simulink library "sm_trackV_lib_terrain_contact"  (R2023b)
settings: Solver=VariableStepAuto  StartTime=0.0  StopTime=10.0  RelTol=1e-3
undefined symbols (not defined in the file): L1, L10, L11, L12, L13, L14, L15, L16, L17, L18, L19, L2, L20, L21, L22, L23, L24, L25, L26, L27, L28, L29, L3, L30, L31, L32, L33, L34, L35, L36, L37, L38, L39, L4, L40, L41, L42, L43, L44, L45, L46, L5, L6, L7, L8, L9, S1, S2, Scene
libraries: $bdroot x141, sm_lib x2
Description:
  | Copyright 2024 The MathWorks, Inc.
settings Model: Creator=smiller  LastModifiedBy=smiller

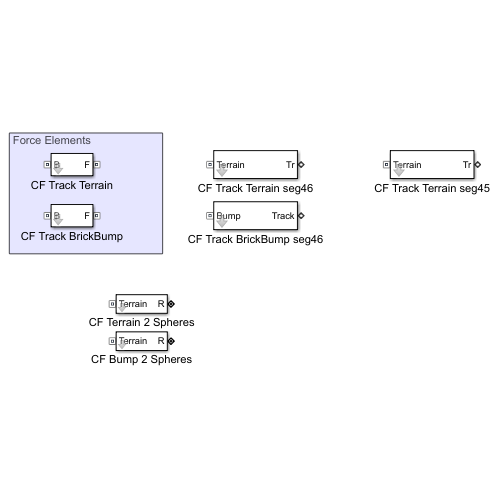
[thumbnail: Simulink's stored preview of the top-level diagram]
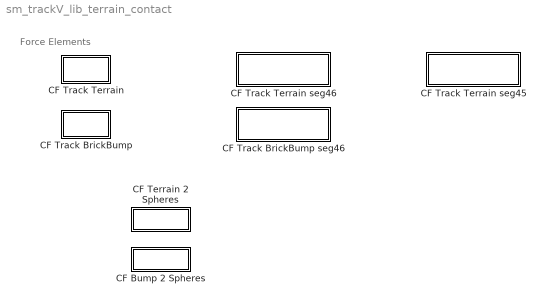
== system sm_trackV_lib_terrain_contact ==
  note: Force Elements
  CF Bump 2 Spheres : Subsystem  mask(Contact Force, Two Spheres to Bump){K_BrickBump=Scene.Contact.BrickBump.K, B_BrickBump=Scene.Contact.BrickBump.B, TW_BrickBump=Scene.Contact.BrickBump.TW, CoefficientOfDynamicFriction=Scene.Contact.Terrain.mud, CoefficientOfStaticFriction=Scene.Contact.Terrain.mus, FrictionalCriticalVelocity=Scene.Contact.Terrain.CV}
      mask prompts: K_BrickBump "Normal Stiffness (N/m)"; B_BrickBump "Normal Damping (N/(m/s))"; TW_BrickBump "Normal Transition Width (m)"; CoefficientOfDynamicFriction "Coefficient of Dynamic Friction"; CoefficientOfStaticFriction "Coefficient of Static Friction"; FrictionalCriticalVelocity "Critical Velocity (m/s)"
      mask help: Models contact force between two spheres and a bump.
      mask TypeOptions K_BrickBump: CF Bump Roller Sphere 1 /NormalStiffness | CF Bump Roller Sphere 2/NormalStiffness
      mask TypeOptions B_BrickBump: CF Bump Roller Sphere 1 /NormalDamping | CF Bump Roller Sphere 2/NormalDamping
      mask TypeOptions TW_BrickBump: CF Bump Roller Sphere 1 /NormalTransitionRegionWidth | CF Bump Roller Sphere 2/NormalTransitionRegionWidth
      mask TypeOptions CoefficientOfDynamicFriction: CF Bump Roller Sphere 1 /CoefficientOfDynamicFriction | CF Bump Roller Sphere 2/CoefficientOfDynamicFriction
      mask TypeOptions CoefficientOfStaticFriction: CF Bump Roller Sphere 1 /CoefficientOfStaticFriction | CF Bump Roller Sphere 2/CoefficientOfStaticFriction
      mask TypeOptions FrictionalCriticalVelocity: CF Bump Roller Sphere 1 /FrictionalCriticalVelocity | CF Bump Roller Sphere 2/FrictionalCriticalVelocity
  CF Terrain 2 Spheres : Subsystem  mask(Contact Force, Two Spheres to Ground){NormalStiffness=Scene.Contact.Spheres.Terrain.K, NormalDamping=Scene.Contact.Spheres.Terrain.B, NormalTransitionRegionWidth=Scene.Contact.Spheres.Terrain.TW, CoefficientOfDynamicFriction=Scene.Contact.Spheres.Terrain.mud, CoefficientOfStaticFriction=Scene.Contact.Spheres.Terrain.mus, FrictionalCriticalVelocity=Scene.Contact.Spheres.Terrain.CV}
      mask prompts: NormalStiffness "Normal Stiffness (N/m)"; NormalDamping "Normal Damping (N/(m/s))"; NormalTransitionRegionWidth "Normal Transition Width (m)"; CoefficientOfDynamicFriction "Coefficient of Dynamic Friction"; CoefficientOfStaticFriction "Coefficient of Static Friction"; FrictionalCriticalVelocity "Critical Velocity (m/s)"
      mask help: Models contact force between two spheres and the ground.
      mask TypeOptions NormalStiffness: CF Roller Sphere Terrain 1/NormalStiffness | CF Roller Sphere Terrain 2/NormalStiffness
      mask TypeOptions NormalDamping: CF Roller Sphere Terrain 1/NormalDamping | CF Roller Sphere Terrain 2/NormalDamping
      mask TypeOptions NormalTransitionRegionWidth: CF Roller Sphere Terrain 1/NormalTransitionRegionWidth | CF Roller Sphere Terrain 2/NormalTransitionRegionWidth
      mask TypeOptions CoefficientOfDynamicFriction: CF Roller Sphere Terrain 1/CoefficientOfDynamicFriction | CF Roller Sphere Terrain 2/CoefficientOfDynamicFriction
      mask TypeOptions CoefficientOfStaticFriction: CF Roller Sphere Terrain 1/CoefficientOfStaticFriction | CF Roller Sphere Terrain 2/CoefficientOfStaticFriction
      mask TypeOptions FrictionalCriticalVelocity: CF Roller Sphere Terrain 1/FrictionalCriticalVelocity | CF Roller Sphere Terrain 2/FrictionalCriticalVelocity
  CF Track BrickBump : Subsystem  mask(Contact Force, Track Segment to Bump){NormalStiffness=Scene.Contact.BrickBump.K, NormalDamping=Scene.Contact.BrickBump.B, NormalTransitionRegionWidth=Scene.Contact.BrickBump.TW}
      mask prompts: NormalStiffness "Normal Stiffness (N/m)"; NormalDamping "Normal Damping (N/(m/s))"; NormalTransitionRegionWidth "Normal Transition Width (m)"
      mask help: Models contact force between a track segment and a bump.
      mask TypeOptions NormalStiffness:
      | Spatial
      | Contact Force/NormalStiffness
      mask TypeOptions NormalDamping:
      | Spatial
      | Contact Force/NormalDamping
      mask TypeOptions NormalTransitionRegionWidth:
      | Spatial
      | Contact Force/NormalTransitionRegionWidth
  CF Track BrickBump seg46 : Subsystem  mask(Contact Forces, Full Track to Bump){K_BrickBump=Scene.Contact.BrickBump.K, B_BrickBump=Scene.Contact.BrickBump.B, TW_BrickBump=Scene.Contact.BrickBump.TW}
      mask prompts: K_BrickBump "Normal Stiffness (N/m)"; B_BrickBump "Normal Damping (N/(m/s))"; TW_BrickBump "Normal Transition Width (m)"
      mask help: Models contact force between all track segments and bump.
  CF Track Terrain : Subsystem  mask(Contact Force, Track Segment to Terrain){NormalStiffness=Scene.Contact.Terrain.K, NormalDamping=Scene.Contact.Terrain.B, NormalTransitionRegionWidth=Scene.Contact.Terrain.TW, CoefficientOfDynamicFriction=Scene.Contact.Terrain.mud, CoefficientOfStaticFriction=Scene.Contact.Terrain.mus, FrictionalCriticalVelocity=Scene.Contact.Terrain.CV}
      mask prompts: NormalStiffness "Normal Stiffness (N/m)"; NormalDamping "Normal Damping (N/(m/s))"; NormalTransitionRegionWidth "Normal Transition Width (m)"; CoefficientOfDynamicFriction "Coefficient of Dynamic Friction"; CoefficientOfStaticFriction "Coefficient of Static Friction"; FrictionalCriticalVelocity "Critical Velocity (m/s)"
      mask help: Models contact force between one track segment and the terrain.
      mask TypeOptions NormalStiffness:
      | Spatial
      | Contact Force/NormalStiffness
      mask TypeOptions NormalDamping:
      | Spatial
      | Contact Force/NormalDamping
      mask TypeOptions NormalTransitionRegionWidth:
      | Spatial
      | Contact Force/NormalTransitionRegionWidth
      mask TypeOptions CoefficientOfDynamicFriction:
      | Spatial
      | Contact Force/CoefficientOfDynamicFriction
      mask TypeOptions CoefficientOfStaticFriction:
      | Spatial
      | Contact Force/CoefficientOfStaticFriction
      mask TypeOptions FrictionalCriticalVelocity:
      | Spatial
      | Contact Force/FrictionalCriticalVelocity
  CF Track Terrain seg45 : Subsystem  mask(Contact Forces, Full Track to Terrain){K_Road=Scene.Contact.Terrain.K, B_Road=Scene.Contact.Terrain.B, TW_Road=Scene.Contact.Terrain.TW, F_dyn_Road=Scene.Contact.Terrain.mud, F_stat_Road=Scene.Contact.Terrain.mus, CV_Road=Scene.Contact.Terrain.CV}
      mask prompts: K_Road "Normal Stiffness (N/m)"; B_Road "Normal Damping (N/(m/s))"; TW_Road "Normal Transition Width (m)"; F_dyn_Road "Coefficient of Dynamic Friction"; F_stat_Road "Coefficient of Static Friction"; CV_Road "Critical Velocity (m/s)"
      mask help: Models contact force between all track segments and the terrain.
  CF Track Terrain seg46 : Subsystem  mask(Contact Forces, Full Track to Terrain){K_Road=Scene.Contact.Terrain.K, B_Road=Scene.Contact.Terrain.B, TW_Road=Scene.Contact.Terrain.TW, F_dyn_Road=Scene.Contact.Terrain.mud, F_stat_Road=Scene.Contact.Terrain.mus, CV_Road=Scene.Contact.Terrain.CV}
      mask prompts: K_Road "Normal Stiffness (N/m)"; B_Road "Normal Damping (N/(m/s))"; TW_Road "Normal Transition Width (m)"; F_dyn_Road "Coefficient of Dynamic Friction"; F_stat_Road "Coefficient of Static Friction"; CV_Road "Critical Velocity (m/s)"
      mask help: Models contact force between all track segments and the terrain.

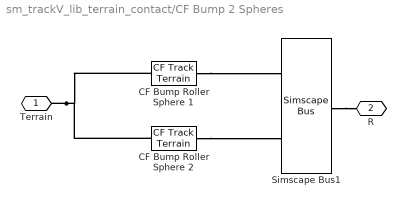
== system sm_trackV_lib_terrain_contact/CF Bump 2 Spheres ==
  "CF Bump Roller Sphere 1 " : $bdroot/CF Track Terrain  NormalStiffness=K_BrickBump  NormalDamping=B_BrickBump  NormalTransitionRegionWidth=TW_BrickBump  CoefficientOfDynamicFriction=CoefficientOfDynamicFriction  CoefficientOfStaticFriction=CoefficientOfStaticFriction  FrictionalCriticalVelocity=FrictionalCriticalVelocity
  CF Bump Roller Sphere 2 : $bdroot/CF Track Terrain  NormalStiffness=K_BrickBump  NormalDamping=B_BrickBump  NormalTransitionRegionWidth=TW_BrickBump  CoefficientOfDynamicFriction=CoefficientOfDynamicFriction  CoefficientOfStaticFriction=CoefficientOfStaticFriction  FrictionalCriticalVelocity=FrictionalCriticalVelocity
  Simscape Bus1 : SimscapeBus  HierarchyStrings=S1;S2
  Terrain : PMIOPort  Side=Left
  R : PMIOPort  Port=2  Side=Right
  connections:
  Simscape Bus1/RConn1 -- R/RConn1
  CF Bump Roller Sphere 2/RConn1 -- Simscape Bus1/LConn2
  Terrain/RConn1 -- CF Bump Roller Sphere 2/LConn1 -- "CF Bump Roller Sphere 1 "/LConn1
  "CF Bump Roller Sphere 1 "/RConn1 -- Simscape Bus1/LConn1

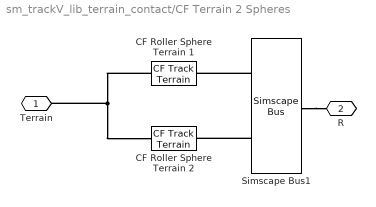
== system sm_trackV_lib_terrain_contact/CF Terrain 2 Spheres ==
  CF Roller Sphere Terrain 1 : $bdroot/CF Track Terrain  NormalStiffness=NormalStiffness  NormalDamping=NormalDamping  NormalTransitionRegionWidth=NormalTransitionRegionWidth  CoefficientOfDynamicFriction=CoefficientOfDynamicFriction  CoefficientOfStaticFriction=CoefficientOfStaticFriction  FrictionalCriticalVelocity=FrictionalCriticalVelocity
  CF Roller Sphere Terrain 2 : $bdroot/CF Track Terrain  NormalStiffness=NormalStiffness  NormalDamping=NormalDamping  NormalTransitionRegionWidth=NormalTransitionRegionWidth  CoefficientOfDynamicFriction=CoefficientOfDynamicFriction  CoefficientOfStaticFriction=CoefficientOfStaticFriction  FrictionalCriticalVelocity=FrictionalCriticalVelocity
  Simscape Bus1 : SimscapeBus  HierarchyStrings=S1;S2
  Terrain : PMIOPort  Side=Left
  R : PMIOPort  Port=2  Side=Right
  connections:
  Simscape Bus1/LConn1 -- CF Roller Sphere Terrain 1/RConn1
  CF Roller Sphere Terrain 1/LConn1 -- CF Roller Sphere Terrain 2/LConn1 -- Terrain/RConn1
  Simscape Bus1/LConn2 -- CF Roller Sphere Terrain 2/RConn1
  Simscape Bus1/RConn1 -- R/RConn1

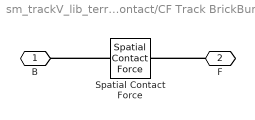
== system sm_trackV_lib_terrain_contact/CF Track BrickBump ==
  Spatial Contact Force : sm_lib/Forces and Torques/Spatial Contact Force  SenseContactBaseRotation=off  SenseContactBaseTranslation=off  CoefficientOfDynamicFriction=0.5  CoefficientOfStaticFriction=0.5  NormalDamping=NormalDamping  NormalDampingUnits=N/(m/s)  SenseContactSignal=off  NormalStiffness=NormalStiffness  NormalStiffnessUnits=N/m  FrictionalCriticalVelocity=1e-3  FrictionalCriticalVelocityUnits=m/s  ZeroCrossDetectContactStartAndEnd=off  SenseContactFollowerRotation=off  SenseContactFollowerTranslation=off  FrictionType=None  SenseFrictionalForceMagnitude=off  SenseNormalForceMagnitude=off  NormalForceType=SmoothSpringDamper  SenseNormalVelocity=off  SensePenetrationDepth=off  SenseSeparationDistance=off  SenseTangentialVelocity=off  NormalTransitionRegionWidth=NormalTransitionRegionWidth  NormalTransitionRegionWidthUnits=m
  B : PMIOPort  Side=Left
  F : PMIOPort  Port=2  Side=Right
  connections:
  F/RConn1 -- Spatial Contact Force/RConn1
  Spatial Contact Force/LConn1 -- B/RConn1

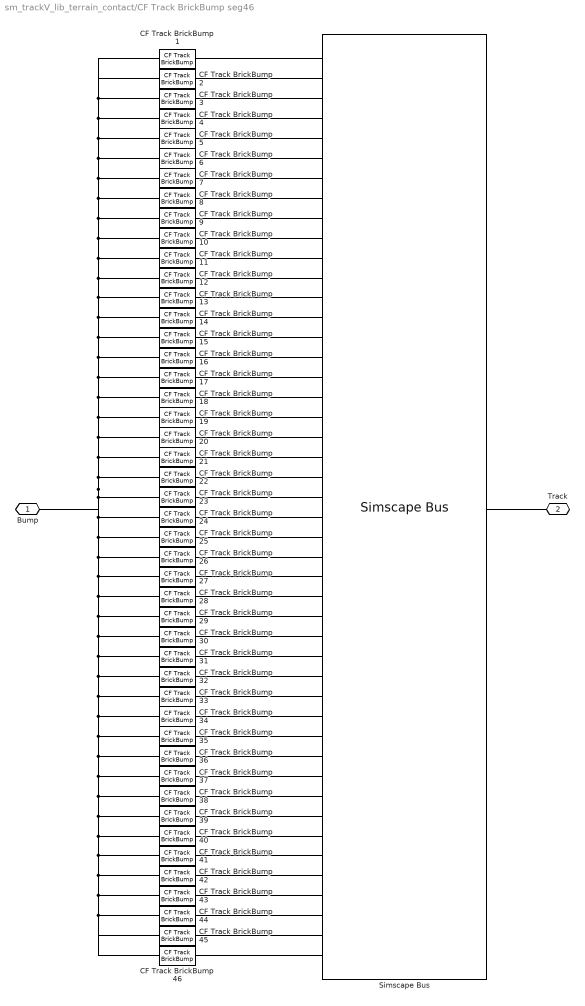
== system sm_trackV_lib_terrain_contact/CF Track BrickBump seg46 ==
  CF Track BrickBump {1..46} (46 alike) : $bdroot/CF Track BrickBump  NormalStiffness=K_BrickBump  NormalDamping=B_BrickBump  NormalTransitionRegionWidth=TW_BrickBump
      settings: LibrarySourceBlock=sm_chain_drive_lib/CF_BrickBump
  Simscape Bus : SimscapeBus  HierarchyStrings=L1;L2;L3;L4;L5;L6;L7;L8;L9;L10;L11;L12;L13;L14;L15;L16;L17;L18;L19;L20;L21;L22;L23;L24;L25;L26;L27;L28;L29;L30;L31;L32;L33;L34;L35;L36;L37;L38;L39;L40;L41;L42;L43;L44;L45;L46  ConnectionType=Bus: CBO_Chain46
  Bump : PMIOPort  Side=Left
  Track : PMIOPort  Port=2  Side=Right
  connections:
  CF Track BrickBump 46/RConn1 -- Simscape Bus/LConn46
  CF Track BrickBump 45/RConn1 -- Simscape Bus/LConn45
  CF Track BrickBump 44/RConn1 -- Simscape Bus/LConn44
  CF Track BrickBump 43/RConn1 -- Simscape Bus/LConn43
  CF Track BrickBump 42/RConn1 -- Simscape Bus/LConn42
  CF Track BrickBump 41/RConn1 -- Simscape Bus/LConn41
  CF Track BrickBump 40/RConn1 -- Simscape Bus/LConn40
  CF Track BrickBump 39/RConn1 -- Simscape Bus/LConn39
  CF Track BrickBump 38/RConn1 -- Simscape Bus/LConn38
  CF Track BrickBump 37/RConn1 -- Simscape Bus/LConn37
  CF Track BrickBump 36/RConn1 -- Simscape Bus/LConn36
  CF Track BrickBump 35/RConn1 -- Simscape Bus/LConn35
  CF Track BrickBump 34/RConn1 -- Simscape Bus/LConn34
  CF Track BrickBump 33/RConn1 -- Simscape Bus/LConn33
  CF Track BrickBump 32/RConn1 -- Simscape Bus/LConn32
  CF Track BrickBump 31/RConn1 -- Simscape Bus/LConn31
  CF Track BrickBump 30/RConn1 -- Simscape Bus/LConn30
  CF Track BrickBump 29/RConn1 -- Simscape Bus/LConn29
  CF Track BrickBump 28/RConn1 -- Simscape Bus/LConn28
  CF Track BrickBump 27/RConn1 -- Simscape Bus/LConn27
  CF Track BrickBump 26/RConn1 -- Simscape Bus/LConn26
  CF Track BrickBump 25/RConn1 -- Simscape Bus/LConn25
  CF Track BrickBump 24/RConn1 -- Simscape Bus/LConn24
  CF Track BrickBump 23/RConn1 -- Simscape Bus/LConn23
  CF Track BrickBump 22/RConn1 -- Simscape Bus/LConn22
  CF Track BrickBump 21/RConn1 -- Simscape Bus/LConn21
  CF Track BrickBump 20/RConn1 -- Simscape Bus/LConn20
  CF Track BrickBump 19/RConn1 -- Simscape Bus/LConn19
  CF Track BrickBump 18/RConn1 -- Simscape Bus/LConn18
  CF Track BrickBump 17/RConn1 -- Simscape Bus/LConn17
  CF Track BrickBump 16/RConn1 -- Simscape Bus/LConn16
  CF Track BrickBump 15/RConn1 -- Simscape Bus/LConn15
  CF Track BrickBump 14/RConn1 -- Simscape Bus/LConn14
  CF Track BrickBump 13/RConn1 -- Simscape Bus/LConn13
  CF Track BrickBump 12/RConn1 -- Simscape Bus/LConn12
  CF Track BrickBump 11/RConn1 -- Simscape Bus/LConn11
  CF Track BrickBump 10/RConn1 -- Simscape Bus/LConn10
  CF Track BrickBump 9/RConn1 -- Simscape Bus/LConn9
  CF Track BrickBump 8/RConn1 -- Simscape Bus/LConn8
  CF Track BrickBump 7/RConn1 -- Simscape Bus/LConn7
  CF Track BrickBump 6/RConn1 -- Simscape Bus/LConn6
  CF Track BrickBump 5/RConn1 -- Simscape Bus/LConn5
  CF Track BrickBump 3/RConn1 -- Simscape Bus/LConn3
  CF Track BrickBump 4/RConn1 -- Simscape Bus/LConn4
  CF Track BrickBump 2/RConn1 -- Simscape Bus/LConn2
  CF Track BrickBump 1/RConn1 -- Simscape Bus/LConn1
  Simscape Bus/RConn1 -- Track/RConn1
  CF Track BrickBump 17/LConn1 -- CF Track BrickBump 18/LConn1 -- CF Track BrickBump 19/LConn1 -- CF Track BrickBump 20/LConn1 -- CF Track BrickBump 21/LConn1 -- CF Track BrickBump 22/LConn1 -- CF Track BrickBump 23/LConn1 -- CF Track BrickBump 24/LConn1 -- CF Track BrickBump 25/LConn1 -- CF Track BrickBump 26/LConn1 -- CF Track BrickBump 27/LConn1 -- CF Track BrickBump 28/LConn1 -- CF Track BrickBump 29/LConn1 -- CF Track BrickBump 30/LConn1 -- CF Track BrickBump 31/LConn1 -- CF Track BrickBump 32/LConn1 -- CF Track BrickBump 33/LConn1 -- CF Track BrickBump 34/LConn1 -- CF Track BrickBump 35/LConn1 -- CF Track BrickBump 36/LConn1 -- CF Track BrickBump 37/LConn1 -- CF Track BrickBump 38/LConn1 -- CF Track BrickBump 39/LConn1 -- CF Track BrickBump 40/LConn1 -- CF Track BrickBump 41/LConn1 -- CF Track BrickBump 42/LConn1 -- CF Track BrickBump 43/LConn1 -- CF Track BrickBump 44/LConn1 -- CF Track BrickBump 46/LConn1 -- CF Track BrickBump 45/LConn1 -- Bump/RConn1 -- CF Track BrickBump 16/LConn1 -- CF Track BrickBump 15/LConn1 -- CF Track BrickBump 14/LConn1 -- CF Track BrickBump 13/LConn1 -- CF Track BrickBump 12/LConn1 -- CF Track BrickBump 11/LConn1 -- CF Track BrickBump 10/LConn1 -- CF Track BrickBump 9/LConn1 -- CF Track BrickBump 8/LConn1 -- CF Track BrickBump 7/LConn1 -- CF Track BrickBump 6/LConn1 -- CF Track BrickBump 5/LConn1 -- CF Track BrickBump 4/LConn1 -- CF Track BrickBump 3/LConn1 -- CF Track BrickBump 2/LConn1 -- CF Track BrickBump 1/LConn1

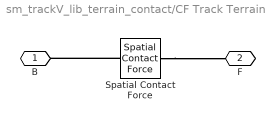
== system sm_trackV_lib_terrain_contact/CF Track Terrain ==
  Spatial Contact Force : sm_lib/Forces and Torques/Spatial Contact Force  SenseContactBaseRotation=off  SenseContactBaseTranslation=off  CoefficientOfDynamicFriction=CoefficientOfDynamicFriction  CoefficientOfStaticFriction=CoefficientOfStaticFriction  NormalDamping=NormalDamping  NormalDampingUnits=N/(m/s)  SenseContactSignal=off  NormalStiffness=NormalStiffness  NormalStiffnessUnits=N/m  FrictionalCriticalVelocity=FrictionalCriticalVelocity  FrictionalCriticalVelocityUnits=m/s  ZeroCrossDetectContactStartAndEnd=off  SenseContactFollowerRotation=off  SenseContactFollowerTranslation=off  FrictionType=SmoothStickSlip  SenseFrictionalForceMagnitude=off  SenseNormalForceMagnitude=off  NormalForceType=SmoothSpringDamper  SenseNormalVelocity=off  SensePenetrationDepth=off  SenseSeparationDistance=off  SenseTangentialVelocity=off  NormalTransitionRegionWidth=NormalTransitionRegionWidth  NormalTransitionRegionWidthUnits=m
  B : PMIOPort  Side=Left
  F : PMIOPort  Port=2  Side=Right
  connections:
  Spatial Contact Force/LConn1 -- B/RConn1
  Spatial Contact Force/RConn1 -- F/RConn1

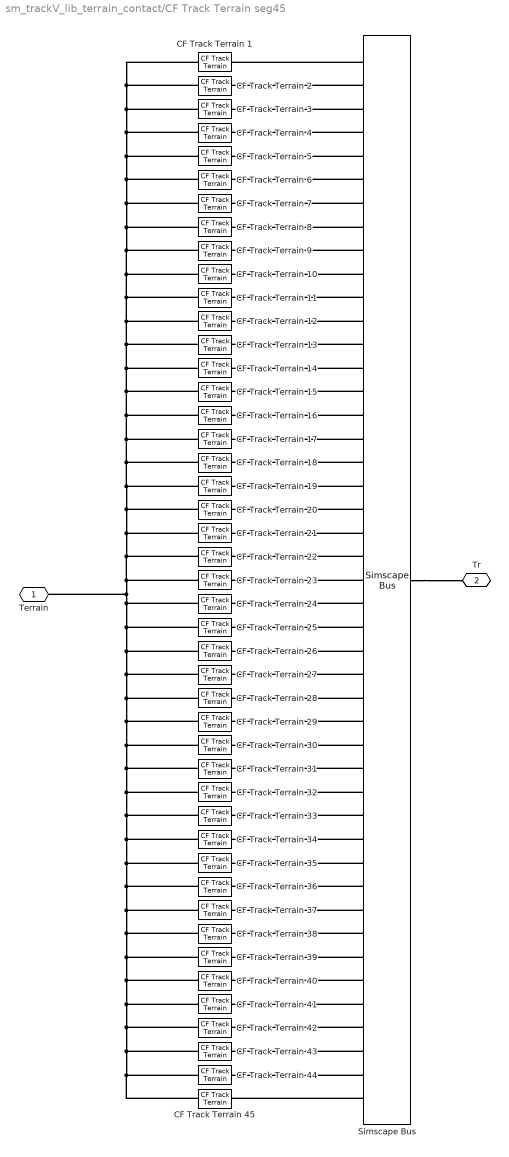
== system sm_trackV_lib_terrain_contact/CF Track Terrain seg45 ==
  CF Track Terrain {1..45} (45 alike) : $bdroot/CF Track Terrain  NormalStiffness=K_Road  NormalDamping=B_Road  NormalTransitionRegionWidth=TW_Road  CoefficientOfDynamicFriction=F_dyn_Road  CoefficientOfStaticFriction=F_stat_Road  FrictionalCriticalVelocity=CV_Road
      settings: LibrarySourceBlock=sm_chain_drive_lib/CF_Road
  Simscape Bus : SimscapeBus  HierarchyStrings=L1;L2;L3;L4;L5;L6;L7;L8;L9;L10;L11;L12;L13;L14;L15;L16;L17;L18;L19;L20;L21;L22;L23;L24;L25;L26;L27;L28;L29;L30;L31;L32;L33;L34;L35;L36;L37;L38;L39;L40;L41;L42;L43;L44;L45  ConnectionType=Bus: CBO_Seg45
  Terrain : PMIOPort  Side=Left
  Tr : PMIOPort  Port=2  Side=Right
  connections:
  Simscape Bus/LConn45 -- CF Track Terrain 45/RConn1
  Simscape Bus/LConn44 -- CF Track Terrain 44/RConn1
  Simscape Bus/LConn43 -- CF Track Terrain 43/RConn1
  Simscape Bus/LConn42 -- CF Track Terrain 42/RConn1
  Simscape Bus/LConn41 -- CF Track Terrain 41/RConn1
  Simscape Bus/LConn40 -- CF Track Terrain 40/RConn1
  Simscape Bus/LConn39 -- CF Track Terrain 39/RConn1
  Simscape Bus/LConn38 -- CF Track Terrain 38/RConn1
  Simscape Bus/LConn37 -- CF Track Terrain 37/RConn1
  Simscape Bus/LConn36 -- CF Track Terrain 36/RConn1
  Simscape Bus/LConn35 -- CF Track Terrain 35/RConn1
  Simscape Bus/LConn34 -- CF Track Terrain 34/RConn1
  Simscape Bus/LConn33 -- CF Track Terrain 33/RConn1
  Simscape Bus/LConn32 -- CF Track Terrain 32/RConn1
  Simscape Bus/LConn31 -- CF Track Terrain 31/RConn1
  Simscape Bus/LConn30 -- CF Track Terrain 30/RConn1
  Simscape Bus/LConn29 -- CF Track Terrain 29/RConn1
  Simscape Bus/LConn28 -- CF Track Terrain 28/RConn1
  Simscape Bus/LConn27 -- CF Track Terrain 27/RConn1
  Simscape Bus/LConn26 -- CF Track Terrain 26/RConn1
  Simscape Bus/LConn25 -- CF Track Terrain 25/RConn1
  Simscape Bus/LConn24 -- CF Track Terrain 24/RConn1
  Simscape Bus/LConn23 -- CF Track Terrain 23/RConn1
  Simscape Bus/LConn22 -- CF Track Terrain 22/RConn1
  Simscape Bus/LConn21 -- CF Track Terrain 21/RConn1
  Simscape Bus/LConn20 -- CF Track Terrain 20/RConn1
  Simscape Bus/LConn19 -- CF Track Terrain 19/RConn1
  Simscape Bus/LConn18 -- CF Track Terrain 18/RConn1
  Simscape Bus/LConn17 -- CF Track Terrain 17/RConn1
  Simscape Bus/LConn16 -- CF Track Terrain 16/RConn1
  Simscape Bus/LConn15 -- CF Track Terrain 15/RConn1
  Simscape Bus/LConn14 -- CF Track Terrain 14/RConn1
  Simscape Bus/LConn13 -- CF Track Terrain 13/RConn1
  Simscape Bus/LConn12 -- CF Track Terrain 12/RConn1
  Simscape Bus/LConn11 -- CF Track Terrain 11/RConn1
  Simscape Bus/LConn10 -- CF Track Terrain 10/RConn1
  Simscape Bus/LConn9 -- CF Track Terrain 9/RConn1
  Simscape Bus/LConn8 -- CF Track Terrain 8/RConn1
  Simscape Bus/LConn7 -- CF Track Terrain 7/RConn1
  Simscape Bus/LConn6 -- CF Track Terrain 6/RConn1
  Simscape Bus/LConn5 -- CF Track Terrain 5/RConn1
  Simscape Bus/LConn3 -- CF Track Terrain 3/RConn1
  Simscape Bus/LConn4 -- CF Track Terrain 4/RConn1
  Simscape Bus/LConn2 -- CF Track Terrain 2/RConn1
  Simscape Bus/LConn1 -- CF Track Terrain 1/RConn1
  Simscape Bus/RConn1 -- Tr/RConn1
  CF Track Terrain 1/LConn1 -- CF Track Terrain 2/LConn1 -- CF Track Terrain 3/LConn1 -- CF Track Terrain 4/LConn1 -- CF Track Terrain 5/LConn1 -- CF Track Terrain 6/LConn1 -- CF Track Terrain 7/LConn1 -- CF Track Terrain 8/LConn1 -- CF Track Terrain 9/LConn1 -- CF Track Terrain 10/LConn1 -- CF Track Terrain 11/LConn1 -- CF Track Terrain 12/LConn1 -- CF Track Terrain 13/LConn1 -- CF Track Terrain 14/LConn1 -- CF Track Terrain 15/LConn1 -- CF Track Terrain 16/LConn1 -- CF Track Terrain 17/LConn1 -- CF Track Terrain 18/LConn1 -- CF Track Terrain 45/LConn1 -- CF Track Terrain 44/LConn1 -- CF Track Terrain 43/LConn1 -- CF Track Terrain 42/LConn1 -- CF Track Terrain 41/LConn1 -- CF Track Terrain 40/LConn1 -- CF Track Terrain 39/LConn1 -- CF Track Terrain 38/LConn1 -- CF Track Terrain 37/LConn1 -- CF Track Terrain 36/LConn1 -- CF Track Terrain 35/LConn1 -- CF Track Terrain 34/LConn1 -- CF Track Terrain 33/LConn1 -- CF Track Terrain 32/LConn1 -- CF Track Terrain 31/LConn1 -- CF Track Terrain 30/LConn1 -- CF Track Terrain 29/LConn1 -- CF Track Terrain 28/LConn1 -- CF Track Terrain 27/LConn1 -- CF Track Terrain 26/LConn1 -- CF Track Terrain 25/LConn1 -- CF Track Terrain 24/LConn1 -- Terrain/RConn1 -- CF Track Terrain 23/LConn1 -- CF Track Terrain 22/LConn1 -- CF Track Terrain 21/LConn1 -- CF Track Terrain 20/LConn1 -- CF Track Terrain 19/LConn1

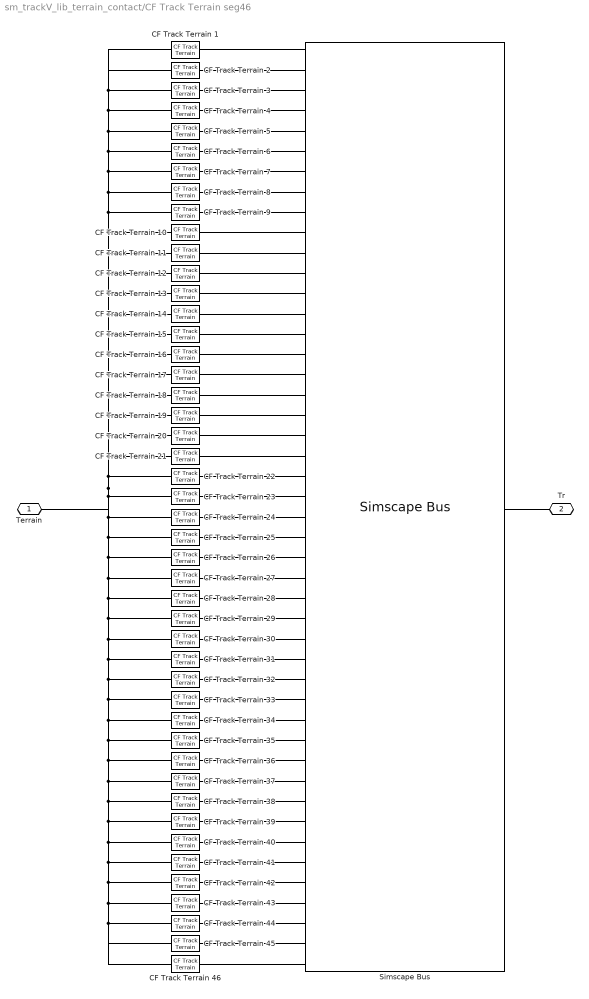
== system sm_trackV_lib_terrain_contact/CF Track Terrain seg46 ==
  CF Track Terrain {1..46} (46 alike) : $bdroot/CF Track Terrain  NormalStiffness=K_Road  NormalDamping=B_Road  NormalTransitionRegionWidth=TW_Road  CoefficientOfDynamicFriction=F_dyn_Road  CoefficientOfStaticFriction=F_stat_Road  FrictionalCriticalVelocity=CV_Road
      settings: LibrarySourceBlock=sm_chain_drive_lib/CF_Road
  Simscape Bus : SimscapeBus  HierarchyStrings=L1;L2;L3;L4;L5;L6;L7;L8;L9;L10;L11;L12;L13;L14;L15;L16;L17;L18;L19;L20;L21;L22;L23;L24;L25;L26;L27;L28;L29;L30;L31;L32;L33;L34;L35;L36;L37;L38;L39;L40;L41;L42;L43;L44;L45;L46  ConnectionType=Bus: CBO_Chain46
  Terrain : PMIOPort  Side=Left
  Tr : PMIOPort  Port=2  Side=Right
  connections:
  CF Track Terrain 19/LConn1 -- CF Track Terrain 20/LConn1 -- CF Track Terrain 21/LConn1 -- CF Track Terrain 22/LConn1 -- CF Track Terrain 23/LConn1 -- Terrain/RConn1 -- CF Track Terrain 24/LConn1 -- CF Track Terrain 25/LConn1 -- CF Track Terrain 26/LConn1 -- CF Track Terrain 27/LConn1 -- CF Track Terrain 28/LConn1 -- CF Track Terrain 29/LConn1 -- CF Track Terrain 30/LConn1 -- CF Track Terrain 31/LConn1 -- CF Track Terrain 32/LConn1 -- CF Track Terrain 33/LConn1 -- CF Track Terrain 34/LConn1 -- CF Track Terrain 35/LConn1 -- CF Track Terrain 36/LConn1 -- CF Track Terrain 37/LConn1 -- CF Track Terrain 38/LConn1 -- CF Track Terrain 39/LConn1 -- CF Track Terrain 40/LConn1 -- CF Track Terrain 41/LConn1 -- CF Track Terrain 42/LConn1 -- CF Track Terrain 43/LConn1 -- CF Track Terrain 44/LConn1 -- CF Track Terrain 46/LConn1 -- CF Track Terrain 45/LConn1 -- CF Track Terrain 18/LConn1 -- CF Track Terrain 17/LConn1 -- CF Track Terrain 16/LConn1 -- CF Track Terrain 15/LConn1 -- CF Track Terrain 14/LConn1 -- CF Track Terrain 13/LConn1 -- CF Track Terrain 12/LConn1 -- CF Track Terrain 11/LConn1 -- CF Track Terrain 10/LConn1 -- CF Track Terrain 9/LConn1 -- CF Track Terrain 8/LConn1 -- CF Track Terrain 7/LConn1 -- CF Track Terrain 6/LConn1 -- CF Track Terrain 5/LConn1 -- CF Track Terrain 4/LConn1 -- CF Track Terrain 3/LConn1 -- CF Track Terrain 2/LConn1 -- CF Track Terrain 1/LConn1
  Simscape Bus/RConn1 -- Tr/RConn1
  Simscape Bus/LConn1 -- CF Track Terrain 1/RConn1
  CF Track Terrain 2/RConn1 -- Simscape Bus/LConn2
  CF Track Terrain 4/RConn1 -- Simscape Bus/LConn4
  CF Track Terrain 3/RConn1 -- Simscape Bus/LConn3
  CF Track Terrain 5/RConn1 -- Simscape Bus/LConn5
  CF Track Terrain 6/RConn1 -- Simscape Bus/LConn6
  CF Track Terrain 7/RConn1 -- Simscape Bus/LConn7
  CF Track Terrain 8/RConn1 -- Simscape Bus/LConn8
  CF Track Terrain 9/RConn1 -- Simscape Bus/LConn9
  CF Track Terrain 10/RConn1 -- Simscape Bus/LConn10
  CF Track Terrain 11/RConn1 -- Simscape Bus/LConn11
  CF Track Terrain 12/RConn1 -- Simscape Bus/LConn12
  CF Track Terrain 13/RConn1 -- Simscape Bus/LConn13
  CF Track Terrain 14/RConn1 -- Simscape Bus/LConn14
  CF Track Terrain 15/RConn1 -- Simscape Bus/LConn15
  CF Track Terrain 16/RConn1 -- Simscape Bus/LConn16
  CF Track Terrain 17/RConn1 -- Simscape Bus/LConn17
  CF Track Terrain 18/RConn1 -- Simscape Bus/LConn18
  CF Track Terrain 19/RConn1 -- Simscape Bus/LConn19
  CF Track Terrain 20/RConn1 -- Simscape Bus/LConn20
  CF Track Terrain 21/RConn1 -- Simscape Bus/LConn21
  CF Track Terrain 22/RConn1 -- Simscape Bus/LConn22
  CF Track Terrain 23/RConn1 -- Simscape Bus/LConn23
  CF Track Terrain 24/RConn1 -- Simscape Bus/LConn24
  CF Track Terrain 25/RConn1 -- Simscape Bus/LConn25
  CF Track Terrain 26/RConn1 -- Simscape Bus/LConn26
  CF Track Terrain 27/RConn1 -- Simscape Bus/LConn27
  CF Track Terrain 28/RConn1 -- Simscape Bus/LConn28
  CF Track Terrain 29/RConn1 -- Simscape Bus/LConn29
  CF Track Terrain 30/RConn1 -- Simscape Bus/LConn30
  CF Track Terrain 31/RConn1 -- Simscape Bus/LConn31
  CF Track Terrain 32/RConn1 -- Simscape Bus/LConn32
  CF Track Terrain 33/RConn1 -- Simscape Bus/LConn33
  CF Track Terrain 34/RConn1 -- Simscape Bus/LConn34
  CF Track Terrain 35/RConn1 -- Simscape Bus/LConn35
  CF Track Terrain 36/RConn1 -- Simscape Bus/LConn36
  CF Track Terrain 37/RConn1 -- Simscape Bus/LConn37
  CF Track Terrain 38/RConn1 -- Simscape Bus/LConn38
  CF Track Terrain 39/RConn1 -- Simscape Bus/LConn39
  CF Track Terrain 40/RConn1 -- Simscape Bus/LConn40
  CF Track Terrain 41/RConn1 -- Simscape Bus/LConn41
  CF Track Terrain 42/RConn1 -- Simscape Bus/LConn42
  CF Track Terrain 43/RConn1 -- Simscape Bus/LConn43
  CF Track Terrain 44/RConn1 -- Simscape Bus/LConn44
  CF Track Terrain 45/RConn1 -- Simscape Bus/LConn45
  CF Track Terrain 46/RConn1 -- Simscape Bus/LConn46
